simulink model "CameraModel"  (R2024b)
settings: Solver=ode4  StartTime=0.0  StopTime=10.0  FixedStep=0.1  RelTol=1e-3
values from neighbouring files (symbols this model uses):
  cx = W/2    (= 512)    [Camera.m]
  cy = H/2    (= 512)    [Camera.m]
  dt = 0.1    [Camera.m]
  f = W/(2*tan(FOV/2))    [Camera.m]
  H = 1024    [Camera.m]
  I = diag([Ix(5), Iy(5), Iz(5)])    [Camera.m]
  Kd_x = Ix * 2 * zeta * wn    [Camera.m]
  Kd_y = Iy * 2 * zeta * wn    [Camera.m]
  Kd_z = Iz * 2 * zeta * wn    [Camera.m]
  Ki_x = 0.0    (= 0)    [Camera.m]
  Ki_y = 0.0    (= 0)    [Camera.m]
  Ki_z = 0.0    (= 0)    [Camera.m]
  Kp_x = Ix * (wn^2)    [Camera.m]
  Kp_y = Iy * (wn^2)    [Camera.m]
  Kp_z = Iz * (wn^2)    [Camera.m]
  P0 = diag([1e-4, 1e-4, 1e-4, 1e-4, 1e-3, 1e-3, 1e-3])    [Camera.m]
  q_0 = eul2quat([yaw, pitch, roll])    [Camera.m]
  R_c = eul2rotm([yaw, pitch, roll])    [Camera.m]
  sigma = 1    [Camera.m]
  stars = [430.226825035 57.6010327889 -649.101965918 -421.510163393 -579.543487823 -810.977245358 -92.8385341278 591.67322486 632.201742584 -349.161737967 930.305422627 -595.811978564 ... (300 elements, 100x3)]    [Starfield_Test.mat]    (also in generateStars.m = [star_x, star_y, star_z])
  W = 1024    [Camera.m]
  w_0 = [0.01, 0.0, 0.0]'    [Camera.m]
undefined symbols (not defined in the file or in its folder): gray, s_intensity
libraries: slpidlib x3, matrix_library x1, vrlib x1
settings Model: Creator=alejandromunozvazquez  LastModifiedBy=alejandromunozvazquez

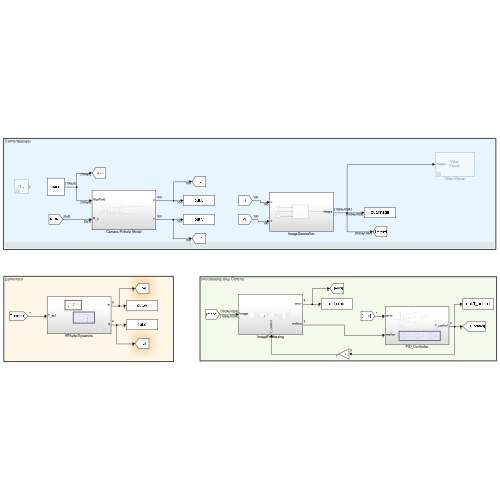
[thumbnail: Simulink's stored preview of the top-level diagram]
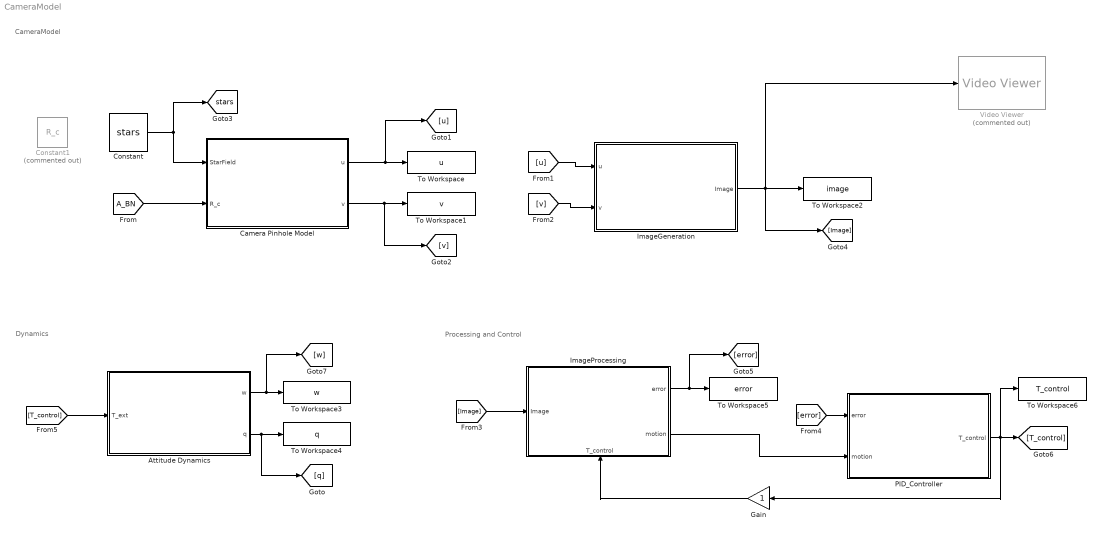
== system CameraModel ==
  note: Processing and Control
  note: Dynamics
  note: CameraModel
  Attitude Dynamics : Subsystem
  Camera Pinhole Model : Subsystem
  Constant : Constant  Value=stars
  Constant1 : Constant  Commented=on  Value=R_c
  Gain : Gain
  ImageGeneration : Subsystem
  ImageProcessing : Subsystem
      settings: PortSchema="{\"entries\":[{\"content\":{\"sides\":[{\"content\":{\"connectorIds\":[\"In1\"]},\"type\":\"ConnectorPlacement.EquallySpacedRectSide\",\"uuid\":\"cefb6310-a581-405a-8101-8623f3d57b98\"},{\"content\":{\"connectorIds\":[\"Out1\",\"Out2\"],\"side\":\"RIGHT\"},\"type\":\"ConnectorPlacement.EquallySpacedRectSide\",\"uuid\":\"16de9d2d-502f-44b2-a135-6b0c6472a31d\"},{\"content\":{\"side\":\"TOP\"},\"type\":\"ConnectorPlacement.EquallySpacedRectSide\",\"uuid\":\"d51e7b6e-a591-4557-adc5-1cc23adf1bf8\"},{\"content\":{\"connectorIds\":[\"In2\"],\"side\":\"BOTTOM\"},\"type\":\"ConnectorPlacement.EquallySpacedRectSide\",\"uuid\":\"ba46090b-2895-4d89-912a-b2ac90d50468\"}]},\"type\":\"ConnectorPlacement.EquallySpacedConnector\",\"uuid\":\"b72943d3-f17b-403e-88fe-0f42ddf20c4f\"}],\"packageUris\":[\"http://schema.mathworks.com/mf0/Connector/R2020b\"],\"version\":\"1.0\"}"
  PID_Controller : Subsystem
  To Workspace : ToWorkspace  VariableName=u  SampleTime=-1
  To Workspace1 : ToWorkspace  VariableName=v  SampleTime=-1
  To Workspace2 : ToWorkspace  VariableName=image  SampleTime=-1
  To Workspace3 : ToWorkspace  VariableName=w  SampleTime=-1
  To Workspace4 : ToWorkspace  VariableName=q  SampleTime=-1
  To Workspace5 : ToWorkspace  VariableName=error  SampleTime=-1
  To Workspace6 : ToWorkspace  VariableName=T_control  SampleTime=-1
  Video Viewer : VideoViewer  Commented=on  colormapValue=gray(256)  FigPos=[336 837 989 604]
  tag scope: stars=global
  wires:
  Attitude Dynamics/1(w) -> [w], To Workspace3/1
  Attitude Dynamics/2(q) -> [q], To Workspace4/1
  Constant/1 -> [stars], Camera Pinhole Model/1(StarField)
  [A_BN] -> Camera Pinhole Model/2(R_c)
  Camera Pinhole Model/1(u) -> [u], To Workspace/1
  Camera Pinhole Model/2(v) -> [v], To Workspace1/1
  [T_control] -> Attitude Dynamics/1(T_ext)
  [u] -> ImageGeneration/1(u)
  [v] -> ImageGeneration/2(v)
  ImageGeneration/1(Image) -> [Image], Video Viewer/1, To Workspace2/1
  [Image] -> ImageProcessing/1(Image)
  ImageProcessing/1(error) -> [error], To Workspace5/1
  [error] -> PID_Controller/1(error)
  PID_Controller/1(T_control) -> Gain/1, [T_control], To Workspace6/1
  ImageProcessing/2(motion) -> PID_Controller/2(motion)
  Gain/1 -> ImageProcessing/2(T_control)

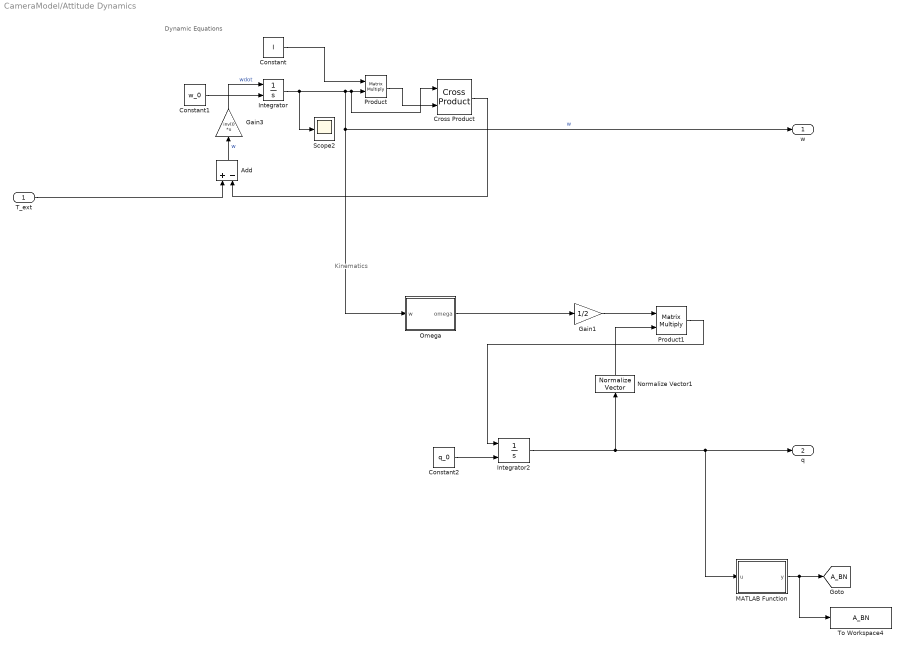
== system CameraModel/Attitude Dynamics ==
  note: Kinematics
  note: Dynamic Equations
  T_ext : Inport
  Add : Sum  Inputs=+-
  Constant : Constant  Value=I
  Constant1 : Constant  Value=w_0
  Constant2 : Constant  Value=q_0
  Cross Product : matrix_library/Cross Product
  Gain1 : Gain  Gain=1/2
  Gain3 : Gain  Gain=inv(I)  Multiplication=Matrix(K*u) (u vector)
  Integrator : Integrator  InitialConditionSource=external
  Integrator2 : Integrator  InitialConditionSource=external
  MATLAB Function : MATLAB Function  TreatAsAtomicUnit=on
  Normalize Vector1 : vrlib/Utilities/Normalize Vector  maxzero=0
  Omega : MATLAB Function  TreatAsAtomicUnit=on
  Product : Product  Multiplication=Matrix(*)
  Product1 : Product  Multiplication=Matrix(*)
  Scope2 : Scope
  To Workspace4 : ToWorkspace  VariableName=A_BN  SampleTime=-1
  w : Outport
  q : Outport  Port=2
  tag scope: A_BN=global
  wires:
  Constant/1 -> Product/1
  Product/1 -> Cross Product/2
  Cross Product/1 -> Add/2
  Integrator/1 -> Scope2/1, Cross Product/1, Product/2, w/1, Omega/1(w)  "w"
  Constant1/1 -> Integrator/2
  T_ext/1 -> Add/1
  Add/1 -> Gain3/1  "w"
  Gain3/1 -> Integrator/1  "wdot"
  Constant2/1 -> Integrator2/2
  Gain1/1 -> Product1/1
  Product1/1 -> Integrator2/1
  Integrator2/1 -> Normalize Vector1/1, MATLAB Function/1(u), q/1
  Normalize Vector1/1 -> Product1/2
  Omega/1(omega) -> Gain1/1
  MATLAB Function/1(y) -> To Workspace4/1, [A_BN]

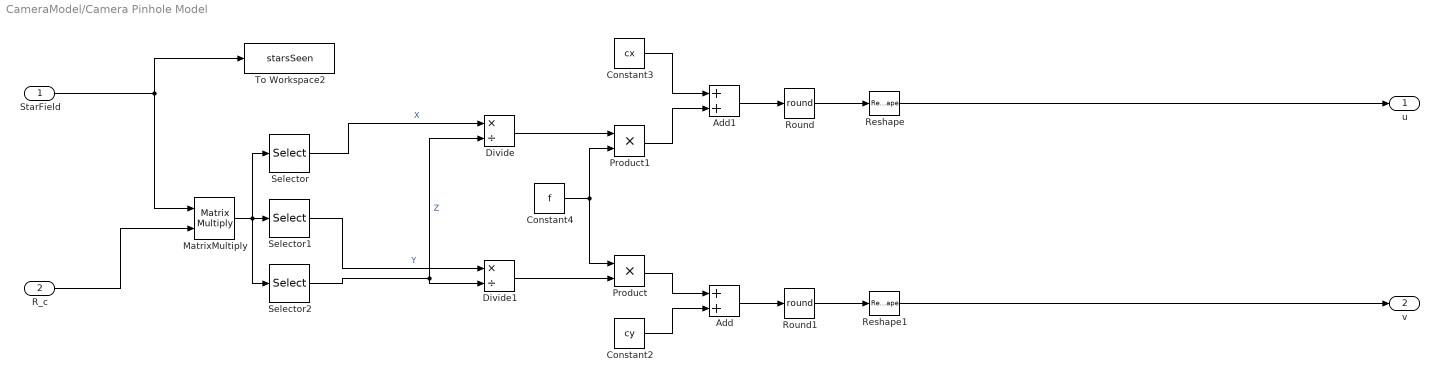
== system CameraModel/Camera Pinhole Model ==
  StarField : Inport
  R_c : Inport  Port=2
  Add : Sum
  Add1 : Sum
  Constant2 : Constant  Value=cy
  Constant3 : Constant  Value=cx
  Constant4 : Constant  Value=f
  Divide : Product  Inputs=*/
  Divide1 : Product  Inputs=*/
  MatrixMultiply : Product  Multiplication=Matrix(*)
  Product : Product
  Product1 : Product
  Reshape : Reshape
  Reshape1 : Reshape
  Round : Rounding  Operator=round
  Round1 : Rounding  Operator=round
  Selector : Selector  NumberOfDimensions=2  InputPortWidth=3  IndexOptions=Select all,Index vector (dialog)  Indices=all,1  OutputSizes=1,1
  Selector1 : Selector  NumberOfDimensions=2  InputPortWidth=3  IndexOptions=Select all,Index vector (dialog)  Indices=all,2  OutputSizes=1,1
  Selector2 : Selector  NumberOfDimensions=2  InputPortWidth=3  IndexOptions=Select all,Index vector (dialog)  Indices=all,3  OutputSizes=1,1
  To Workspace2 : ToWorkspace  VariableName=starsSeen  SampleTime=-1
  u : Outport
  v : Outport  Port=2
  wires:
  Constant2/1 -> Add/2
  R_c/1 -> MatrixMultiply/2
  Round/1 -> Reshape/1
  Divide/1 -> Product1/1
  Product/1 -> Add/1
  Add/1 -> Round1/1
  Selector/1 -> Divide/1  "X"
  Selector1/1 -> Divide1/1  "Y"
  Selector2/1 -> Divide1/2, Divide/2  "Z"
  Add1/1 -> Round/1
  Round1/1 -> Reshape1/1
  MatrixMultiply/1 -> Selector2/1, Selector1/1, Selector/1
  Constant4/1 -> Product/1, Product1/2
  StarField/1 -> MatrixMultiply/1, To Workspace2/1
  Divide1/1 -> Product/2
  Product1/1 -> Add1/2
  Constant3/1 -> Add1/1
  Reshape/1 -> u/1
  Reshape1/1 -> v/1

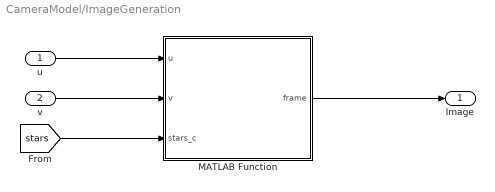
== system CameraModel/ImageGeneration ==
  u : Inport
  v : Inport  Port=2
  MATLAB Function : MATLAB Function  TreatAsAtomicUnit=on
  Image : Outport
  wires:
  u/1 -> MATLAB Function/1(u)
  v/1 -> MATLAB Function/2(v)
  [stars] -> MATLAB Function/3(stars_c)
  MATLAB Function/1(frame) -> Image/1

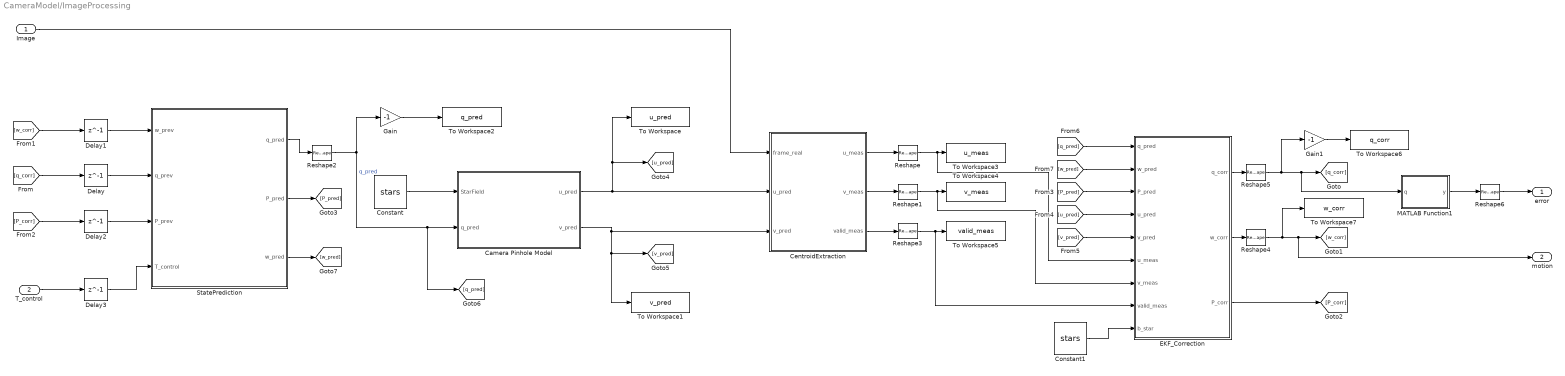
== system CameraModel/ImageProcessing ==
  Image : Inport
  T_control : Inport  Port=2
  Camera Pinhole Model : Subsystem
  CentroidExtraction : MATLAB Function  TreatAsAtomicUnit=on
  Constant : Constant  Value=stars
  Constant1 : Constant  Value=stars
  Delay : Delay  DelayLength=1  InitialCondition=q_0
  Delay1 : Delay  DelayLength=1  InitialCondition=w_0
  Delay2 : Delay  DelayLength=1  InitialCondition=P0
  Delay3 : Delay  DelayLength=1  InitialCondition=[0;0;0]
  EKF_Correction : MATLAB Function  TreatAsAtomicUnit=on
  Gain : Gain  Gain=-1
  Gain1 : Gain  Gain=-1
  MATLAB Function1 : MATLAB Function  TreatAsAtomicUnit=on
  Reshape{,1..6} (7 alike) : Reshape
  StatePrediction : MATLAB Function  TreatAsAtomicUnit=on
  To Workspace : ToWorkspace  VariableName=u_pred  SampleTime=-1
  To Workspace1 : ToWorkspace  VariableName=v_pred  SampleTime=-1
  To Workspace2 : ToWorkspace  VariableName=q_pred  SampleTime=-1
  To Workspace3 : ToWorkspace  VariableName=u_meas  SampleTime=-1
  To Workspace4 : ToWorkspace  VariableName=v_meas  SampleTime=-1
  To Workspace5 : ToWorkspace  VariableName=valid_meas  SampleTime=-1
  To Workspace6 : ToWorkspace  VariableName=q_corr  SampleTime=-1
  To Workspace7 : ToWorkspace  VariableName=w_corr  SampleTime=-1
  error : Outport
  motion : Outport  Port=2
  wires:
  Image/1 -> CentroidExtraction/1(frame_real)
  Delay/1 -> StatePrediction/2(q_prev)
  Delay1/1 -> StatePrediction/1(w_prev)
  StatePrediction/1(q_pred) -> Reshape2/1
  Reshape2/1 -> Gain/1, [q_pred], Camera Pinhole Model/2(q_pred)  "q_pred"
  Constant/1 -> Camera Pinhole Model/1(StarField)
  Camera Pinhole Model/1(u_pred) -> CentroidExtraction/2(u_pred), [u_pred], To Workspace/1
  CentroidExtraction/1(u_meas) -> Reshape/1
  CentroidExtraction/2(v_meas) -> Reshape1/1
  Reshape/1 -> EKF_Correction/6(u_meas), To Workspace3/1
  Reshape1/1 -> EKF_Correction/7(v_meas), To Workspace4/1
  CentroidExtraction/3(valid_meas) -> Reshape3/1
  Reshape3/1 -> EKF_Correction/8(valid_meas), To Workspace5/1
  EKF_Correction/1(q_corr) -> Reshape5/1
  EKF_Correction/3(P_corr) -> [P_corr]
  EKF_Correction/2(w_corr) -> Reshape4/1
  [q_corr] -> Delay/1
  [w_corr] -> Delay1/1
  [P_corr] -> Delay2/1
  Delay2/1 -> StatePrediction/3(P_prev)
  StatePrediction/2(P_pred) -> [P_pred]
  [P_pred] -> EKF_Correction/3(P_pred)
  Constant1/1 -> EKF_Correction/9(b_star)
  Camera Pinhole Model/2(v_pred) -> [v_pred], To Workspace1/1, CentroidExtraction/3(v_pred)
  [v_pred] -> EKF_Correction/5(v_pred)
  [u_pred] -> EKF_Correction/4(u_pred)
  [q_pred] -> EKF_Correction/1(q_pred)
  [w_pred] -> EKF_Correction/2(w_pred)
  StatePrediction/3(w_pred) -> [w_pred]
  Reshape4/1 -> To Workspace7/1, motion/1, [w_corr]
  Reshape5/1 -> Gain1/1, MATLAB Function1/1(q), [q_corr]
  MATLAB Function1/1(y) -> Reshape6/1
  Reshape6/1 -> error/1
  T_control/1 -> Delay3/1
  Delay3/1 -> StatePrediction/4(T_control)
  Gain/1 -> To Workspace2/1
  Gain1/1 -> To Workspace6/1

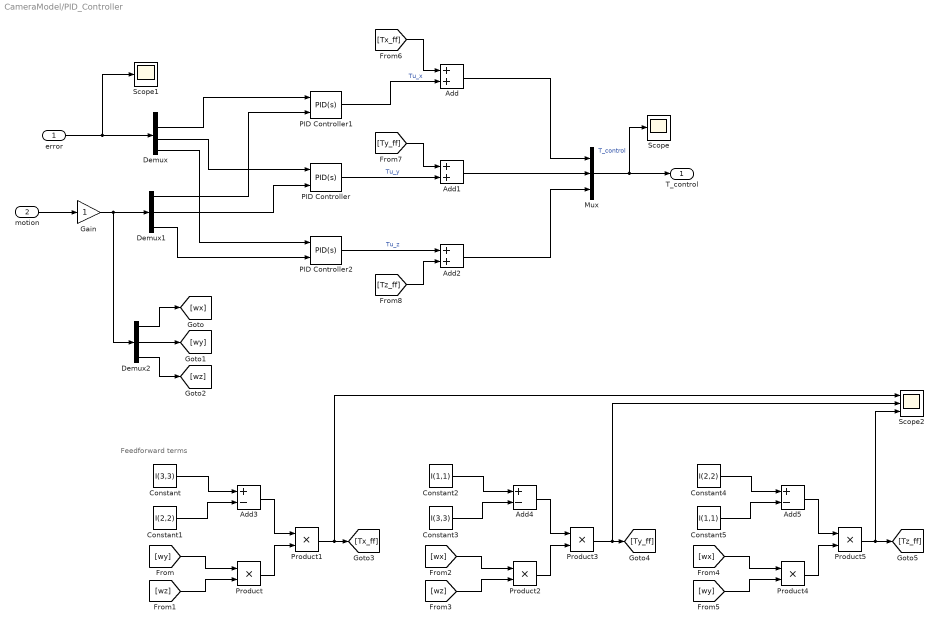
== system CameraModel/PID_Controller ==
  note: Feedforward terms
  error : Inport
  motion : Inport  Port=2
  Add : Sum
  Add1 : Sum
  Add2 : Sum
  Add3 : Sum  Inputs=+-
  Add4 : Sum  Inputs=+-
  Add5 : Sum  Inputs=+-
  Constant : Constant  Value=I(3,3)
  Constant1 : Constant  Value=I(2,2)
  Constant2 : Constant  Value=I(1,1)
  Constant3 : Constant  Value=I(3,3)
  Constant4 : Constant  Value=I(2,2)
  Constant5 : Constant  Value=I(1,1)
  Demux : Demux
  Demux1 : Demux  Outputs=3
  Demux2 : Demux  Outputs=3
  Gain : Gain
  Mux : Mux  Inputs=3
  PID Controller : slpidlib/PID Controller  Controller=PID  Form=Parallel  TimeDomain=Continuous-time  UseExternalTs=off  SampleTime=-1  IntegratorMethod=Forward Euler  FilterMethod=Forward Euler  ControllerParametersSource=internal  P=Kp_y  I=Ki_y  UseKiTs=off  D=Kd_y  UseExternalDerivativeSource=on  N=10  UseFilter=on  TunerSelectOption=Transfer Function Based (PID Tuner App)  InitialConditionSource=internal  InitialConditionForIntegrator=0  InitialConditionForFilter=0  DifferentiatorICPrevScaledInput=0  ExternalReset=none  TrackingMode=off  Kt=1  LimitOutput=off  SatLimitsSource=internal  UpperSaturationLimit=inf  LowerSaturationLimit=-inf  LinearizeAsGain=on  AntiWindupMode=none  Kb=1  LimitIntegrator=off  UpperIntegratorSaturationLimit=inf  LowerIntegratorSaturationLimit=-inf  POutMin=[]  POutMax=[]  IOutMin=[]  IOutMax=[]  DOutMin=[]  DOutMax=[]  NOutMin=[]  NOutMax=[]  SumOutMin=[]  SumOutMax=[]  SaturationOutMin=[]  SaturationOutMax=[]  PParamMin=[]  PParamMax=[]  IParamMin=[]  IParamMax=[]  DParamMin=[]  DParamMax=[]  NParamMin=[]  NParamMax=[]  KbParamMin=[]  KbParamMax=[]  KtParamMin=[]  KtParamMax=[]  KbOutMin=[]  KbOutMax=[]  KtOutMin=[]  KtOutMax=[]  IntegratorOutMin=[]  IntegratorOutMax=[]  FilterOutMin=[]  FilterOutMax=[]  SumI1OutMin=[]  SumI1OutMax=[]  SumI2OutMin=[]  SumI2OutMax=[]  SumI3OutMin=[]  SumI3OutMax=[]  SumI4OutMin=[]  SumI4OutMax=[]  SumDOutMin=[]  SumDOutMax=[]  DifferentiatorOutMin=[]  DifferentiatorOutMax=[]  FilterDiffOutCoefMin=[]  FilterDiffOutCoefMax=[]  ReciprocalOutMin=[]  ReciprocalOutMax=[]  SumDenOutMin=[]  SumDenOutMax=[]  SumNumOutMin=[]  SumNumOutMax=[]  DivideOutMin=[]  DivideOutMax=[]  UdiffTsProdOutMin=[]  UdiffTsProdOutMax=[]  NTsProdOutMin=[]  NTsProdOutMax=[]  UintegralTsProdOutMin=[]  UintegralTsProdOutMax=[]  UngainTsProdOutMin=[]  UngainTsProdOutMax=[]  ClampingZeroOutDataTypeStr=Inherit: Inherit via back propagation  ClampingZeroOutMin=[]  ClampingZeroOutMax=[]  FilterDenConstantOutDataTypeStr=Inherit: Inherit via back propagation  FilterDenConstantOutMin=[]  FilterDenConstantOutMax=[]  PCopyOutDataTypeStr=Inherit: Inherit via back propagation  PCopyOutMin=[]  PCopyOutMax=[]  NCopyOutDataTypeStr=Inherit: Inherit via back propagation  NCopyOutMin=[]  NCopyOutMax=[]  IntegratorContinuousStateAttributes=''  IntegratorStateMustResolveToSignalObject=off  IntegratorRTWStateStorageClass=Auto  FilterContinuousStateAttributes=''  FilterStateMustResolveToSignalObject=off  FilterRTWStateStorageClass=Auto  ParallelPVariant=InternalParameters  IdealPVariant=Disabled  IVariant=InternalParameters  DVariant=InternalParameters  IntegratorVariant=Continuous  SatVariant=Disabled  AWVariant=Passthrough  PCopyVariant=Disabled  TRVariant=Disabled  FdbkBlocksVariant=Forward  IdealPFdbkVariant=Disabled  SatFdbkVariant=Disabled  DerivativeFilterVariant=ContFilterOnly  NVariant=InternalParameters  NCopyVariant=Disabled  FilterICVariant=InternalICsFilter  IntegratorICVariant=InternalICs  ExternalResetVariant=Disabled  TRSumVariant=Passthrough  SumFdbkVariant=Disabled  SumVariant=Sum_PID  TsampFilterVariant=InternalTs  TsampNgainVariant=Passthrough  TsampIntegralVariant=Disabled_SignalSpec  ExternalSaturationOutDataTypeStr=Inherit: Same as second input  DerivativeSourceVariant=ExternalYdot  PreIntVariant=InternalPreInt
  PID Controller1 : slpidlib/PID Controller  Controller=PID  Form=Parallel  TimeDomain=Continuous-time  UseExternalTs=off  SampleTime=-1  IntegratorMethod=Forward Euler  FilterMethod=Forward Euler  ControllerParametersSource=internal  P=Kp_x  I=Ki_x  UseKiTs=off  D=Kd_x  UseExternalDerivativeSource=on  N=10  UseFilter=on  TunerSelectOption=Transfer Function Based (PID Tuner App)  InitialConditionSource=internal  InitialConditionForIntegrator=0  InitialConditionForFilter=0  DifferentiatorICPrevScaledInput=0  ExternalReset=none  TrackingMode=off  Kt=1  LimitOutput=off  SatLimitsSource=internal  UpperSaturationLimit=inf  LowerSaturationLimit=-inf  LinearizeAsGain=on  AntiWindupMode=none  Kb=1  LimitIntegrator=off  UpperIntegratorSaturationLimit=inf  LowerIntegratorSaturationLimit=-inf  POutMin=[]  POutMax=[]  IOutMin=[]  IOutMax=[]  DOutMin=[]  DOutMax=[]  NOutMin=[]  NOutMax=[]  SumOutMin=[]  SumOutMax=[]  SaturationOutMin=[]  SaturationOutMax=[]  PParamMin=[]  PParamMax=[]  IParamMin=[]  IParamMax=[]  DParamMin=[]  DParamMax=[]  NParamMin=[]  NParamMax=[]  KbParamMin=[]  KbParamMax=[]  KtParamMin=[]  KtParamMax=[]  KbOutMin=[]  KbOutMax=[]  KtOutMin=[]  KtOutMax=[]  IntegratorOutMin=[]  IntegratorOutMax=[]  FilterOutMin=[]  FilterOutMax=[]  SumI1OutMin=[]  SumI1OutMax=[]  SumI2OutMin=[]  SumI2OutMax=[]  SumI3OutMin=[]  SumI3OutMax=[]  SumI4OutMin=[]  SumI4OutMax=[]  SumDOutMin=[]  SumDOutMax=[]  DifferentiatorOutMin=[]  DifferentiatorOutMax=[]  FilterDiffOutCoefMin=[]  FilterDiffOutCoefMax=[]  ReciprocalOutMin=[]  ReciprocalOutMax=[]  SumDenOutMin=[]  SumDenOutMax=[]  SumNumOutMin=[]  SumNumOutMax=[]  DivideOutMin=[]  DivideOutMax=[]  UdiffTsProdOutMin=[]  UdiffTsProdOutMax=[]  NTsProdOutMin=[]  NTsProdOutMax=[]  UintegralTsProdOutMin=[]  UintegralTsProdOutMax=[]  UngainTsProdOutMin=[]  UngainTsProdOutMax=[]  ClampingZeroOutDataTypeStr=Inherit: Inherit via back propagation  ClampingZeroOutMin=[]  ClampingZeroOutMax=[]  FilterDenConstantOutDataTypeStr=Inherit: Inherit via back propagation  FilterDenConstantOutMin=[]  FilterDenConstantOutMax=[]  PCopyOutDataTypeStr=Inherit: Inherit via back propagation  PCopyOutMin=[]  PCopyOutMax=[]  NCopyOutDataTypeStr=Inherit: Inherit via back propagation  NCopyOutMin=[]  NCopyOutMax=[]  IntegratorContinuousStateAttributes=''  IntegratorStateMustResolveToSignalObject=off  IntegratorRTWStateStorageClass=Auto  FilterContinuousStateAttributes=''  FilterStateMustResolveToSignalObject=off  FilterRTWStateStorageClass=Auto  ParallelPVariant=InternalParameters  IdealPVariant=Disabled  IVariant=InternalParameters  DVariant=InternalParameters  IntegratorVariant=Continuous  SatVariant=Disabled  AWVariant=Passthrough  PCopyVariant=Disabled  TRVariant=Disabled  FdbkBlocksVariant=Forward  IdealPFdbkVariant=Disabled  SatFdbkVariant=Disabled  DerivativeFilterVariant=ContFilterOnly  NVariant=InternalParameters  NCopyVariant=Disabled  FilterICVariant=InternalICsFilter  IntegratorICVariant=InternalICs  ExternalResetVariant=Disabled  TRSumVariant=Passthrough  SumFdbkVariant=Disabled  SumVariant=Sum_PID  TsampFilterVariant=InternalTs  TsampNgainVariant=Passthrough  TsampIntegralVariant=Disabled_SignalSpec  ExternalSaturationOutDataTypeStr=Inherit: Same as second input  DerivativeSourceVariant=ExternalYdot  PreIntVariant=InternalPreInt
  PID Controller2 : slpidlib/PID Controller  Controller=PID  Form=Parallel  TimeDomain=Continuous-time  UseExternalTs=off  SampleTime=-1  IntegratorMethod=Forward Euler  FilterMethod=Forward Euler  ControllerParametersSource=internal  P=Kp_z  I=Ki_z  UseKiTs=off  D=Kd_z  UseExternalDerivativeSource=on  N=10  UseFilter=on  TunerSelectOption=Transfer Function Based (PID Tuner App)  InitialConditionSource=internal  InitialConditionForIntegrator=0  InitialConditionForFilter=0  DifferentiatorICPrevScaledInput=0  ExternalReset=none  TrackingMode=off  Kt=1  LimitOutput=off  SatLimitsSource=internal  UpperSaturationLimit=inf  LowerSaturationLimit=-inf  LinearizeAsGain=on  AntiWindupMode=none  Kb=1  LimitIntegrator=off  UpperIntegratorSaturationLimit=inf  LowerIntegratorSaturationLimit=-inf  POutMin=[]  POutMax=[]  IOutMin=[]  IOutMax=[]  DOutMin=[]  DOutMax=[]  NOutMin=[]  NOutMax=[]  SumOutMin=[]  SumOutMax=[]  SaturationOutMin=[]  SaturationOutMax=[]  PParamMin=[]  PParamMax=[]  IParamMin=[]  IParamMax=[]  DParamMin=[]  DParamMax=[]  NParamMin=[]  NParamMax=[]  KbParamMin=[]  KbParamMax=[]  KtParamMin=[]  KtParamMax=[]  KbOutMin=[]  KbOutMax=[]  KtOutMin=[]  KtOutMax=[]  IntegratorOutMin=[]  IntegratorOutMax=[]  FilterOutMin=[]  FilterOutMax=[]  SumI1OutMin=[]  SumI1OutMax=[]  SumI2OutMin=[]  SumI2OutMax=[]  SumI3OutMin=[]  SumI3OutMax=[]  SumI4OutMin=[]  SumI4OutMax=[]  SumDOutMin=[]  SumDOutMax=[]  DifferentiatorOutMin=[]  DifferentiatorOutMax=[]  FilterDiffOutCoefMin=[]  FilterDiffOutCoefMax=[]  ReciprocalOutMin=[]  ReciprocalOutMax=[]  SumDenOutMin=[]  SumDenOutMax=[]  SumNumOutMin=[]  SumNumOutMax=[]  DivideOutMin=[]  DivideOutMax=[]  UdiffTsProdOutMin=[]  UdiffTsProdOutMax=[]  NTsProdOutMin=[]  NTsProdOutMax=[]  UintegralTsProdOutMin=[]  UintegralTsProdOutMax=[]  UngainTsProdOutMin=[]  UngainTsProdOutMax=[]  ClampingZeroOutDataTypeStr=Inherit: Inherit via back propagation  ClampingZeroOutMin=[]  ClampingZeroOutMax=[]  FilterDenConstantOutDataTypeStr=Inherit: Inherit via back propagation  FilterDenConstantOutMin=[]  FilterDenConstantOutMax=[]  PCopyOutDataTypeStr=Inherit: Inherit via back propagation  PCopyOutMin=[]  PCopyOutMax=[]  NCopyOutDataTypeStr=Inherit: Inherit via back propagation  NCopyOutMin=[]  NCopyOutMax=[]  IntegratorContinuousStateAttributes=''  IntegratorStateMustResolveToSignalObject=off  IntegratorRTWStateStorageClass=Auto  FilterContinuousStateAttributes=''  FilterStateMustResolveToSignalObject=off  FilterRTWStateStorageClass=Auto  ParallelPVariant=InternalParameters  IdealPVariant=Disabled  IVariant=InternalParameters  DVariant=InternalParameters  IntegratorVariant=Continuous  SatVariant=Disabled  AWVariant=Passthrough  PCopyVariant=Disabled  TRVariant=Disabled  FdbkBlocksVariant=Forward  IdealPFdbkVariant=Disabled  SatFdbkVariant=Disabled  DerivativeFilterVariant=ContFilterOnly  NVariant=InternalParameters  NCopyVariant=Disabled  FilterICVariant=InternalICsFilter  IntegratorICVariant=InternalICs  ExternalResetVariant=Disabled  TRSumVariant=Passthrough  SumFdbkVariant=Disabled  SumVariant=Sum_PID  TsampFilterVariant=InternalTs  TsampNgainVariant=Passthrough  TsampIntegralVariant=Disabled_SignalSpec  ExternalSaturationOutDataTypeStr=Inherit: Same as second input  DerivativeSourceVariant=ExternalYdot  PreIntVariant=InternalPreInt
  Product{,1..5} (6 alike) : Product
  Scope : Scope
  Scope1 : Scope
  Scope2 : Scope  NumInputPorts=3
  T_control : Outport
  wires:
  error/1 -> Scope1/1, Demux/1
  Demux/3 -> PID Controller/1
  Demux/2 -> PID Controller1/1
  PID Controller/1 -> Add1/2  "Tu_y"
  PID Controller1/1 -> Add/2  "Tu_x"
  Demux/4 -> PID Controller2/1
  PID Controller2/1 -> Add2/1  "Tu_z"
  Mux/1 -> T_control/1, Scope/1  "T_control"
  motion/1 -> Gain/1
  Demux1/1 -> PID Controller1/2
  Gain/1 -> Demux2/1, Demux1/1
  Demux1/3 -> PID Controller2/2
  Demux1/2 -> PID Controller/2
  Demux2/1 -> [wx]
  Demux2/2 -> [wy]
  Demux2/3 -> [wz]
  Constant1/1 -> Add3/2
  Constant/1 -> Add3/1
  [wy] -> Product/1
  [wz] -> Product/2
  Add3/1 -> Product1/1
  Product/1 -> Product1/2
  Product1/1 -> Scope2/1, [Tx_ff]
  Product3/1 -> Scope2/2, [Ty_ff]
  Product2/1 -> Product3/2
  Add4/1 -> Product3/1
  [wz] -> Product2/2
  [wx] -> Product2/1
  Constant2/1 -> Add4/1
  Constant3/1 -> Add4/2
  Constant5/1 -> Add5/2
  Constant4/1 -> Add5/1
  [wx] -> Product4/1
  [wy] -> Product4/2
  Add5/1 -> Product5/1
  Product4/1 -> Product5/2
  Product5/1 -> Scope2/3, [Tz_ff]
  [Tx_ff] -> Add/1
  [Ty_ff] -> Add1/1
  [Tz_ff] -> Add2/2
  Add/1 -> Mux/1
  Add1/1 -> Mux/2
  Add2/1 -> Mux/3

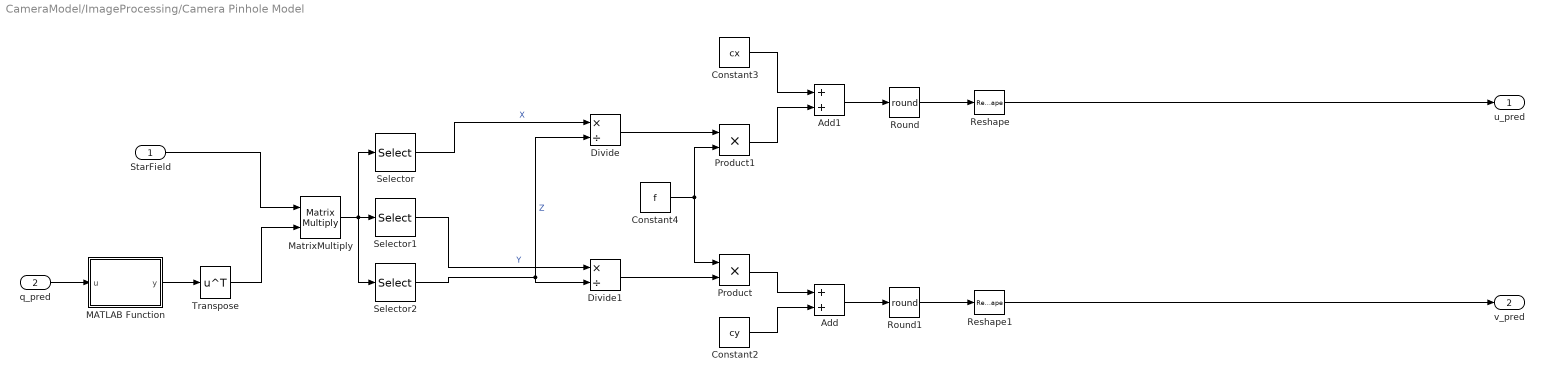
== system CameraModel/ImageProcessing/Camera Pinhole Model ==
  StarField : Inport
  q_pred : Inport  Port=2
  Add : Sum
  Add1 : Sum
  Constant2 : Constant  Value=cy
  Constant3 : Constant  Value=cx
  Constant4 : Constant  Value=f
  Divide : Product  Inputs=*/
  Divide1 : Product  Inputs=*/
  MATLAB Function : MATLAB Function  TreatAsAtomicUnit=on
  MatrixMultiply : Product  Multiplication=Matrix(*)
  Product : Product
  Product1 : Product
  Reshape : Reshape
  Reshape1 : Reshape
  Round : Rounding  Operator=round
  Round1 : Rounding  Operator=round
  Selector : Selector  NumberOfDimensions=2  InputPortWidth=3  IndexOptions=Select all,Index vector (dialog)  Indices=all,1  OutputSizes=1,1
  Selector1 : Selector  NumberOfDimensions=2  InputPortWidth=3  IndexOptions=Select all,Index vector (dialog)  Indices=all,2  OutputSizes=1,1
  Selector2 : Selector  NumberOfDimensions=2  InputPortWidth=3  IndexOptions=Select all,Index vector (dialog)  Indices=all,3  OutputSizes=1,1
  Transpose : Math  Operator=transpose
  u_pred : Outport
  v_pred : Outport  Port=2
  wires:
  Constant2/1 -> Add/2
  q_pred/1 -> MATLAB Function/1(u)
  Round/1 -> Reshape/1
  Divide/1 -> Product1/1
  Product/1 -> Add/1
  Add/1 -> Round1/1
  Selector/1 -> Divide/1  "X"
  Selector1/1 -> Divide1/1  "Y"
  Selector2/1 -> Divide1/2, Divide/2  "Z"
  Add1/1 -> Round/1
  Round1/1 -> Reshape1/1
  MatrixMultiply/1 -> Selector2/1, Selector1/1, Selector/1
  Constant4/1 -> Product/1, Product1/2
  StarField/1 -> MatrixMultiply/1
  Divide1/1 -> Product/2
  Product1/1 -> Add1/2
  Constant3/1 -> Add1/1
  Reshape/1 -> u_pred/1
  Reshape1/1 -> v_pred/1
  MATLAB Function/1(y) -> Transpose/1
  Transpose/1 -> MatrixMultiply/2

== matlab function CameraModel/ImageProcessing/MATLAB Function1 ==
  data: q input; y output; q_0 parameter
function y = fcn(q, q_0)

    q_0 = q_0(:) / norm(q_0);
    q   = q(:)   / norm(q);

    % Inverso = conjugado para cuaterniones unitarios
    q_inv = [q_0(1); -q_0(2); -q_0(3); -q_0(4)];

    % Producto cuaterniónico manual: q_err = q_inv ⊗ q
    % Convenio [w, x, y, z]
    w1=q_inv(1); x1=q_inv(2); y1=q_inv(3); z1=q_inv(4);
    w2=q(1);     x2=q(2);     y2=q(3);     z2=q(4);

    q_err = [ w1*w2 - x1*x2 - y1*y2 - z1*z2;
              w1*x2 + x1*w2 + y1*z2 - z1*y2;
              w1*y2 - x1*z2 + y1*w2 + z1*x2;
              w1*z2 + x1*y2 - y1*x2 + z1*w2 ];

    % Ángulos de Euler del error
    %y = quat2eul(q_err');
    y = [q_err(1); q_err(2); q_err(3); q_err(4)];
end

== matlab function CameraModel/Attitude Dynamics/Omega ==
  data: w input; omega output size=[4,4]
function omega = fcn(w)

omega = zeros(4,4);
wx = w(1);
wy = w(2);
wz = w(3);



omega = [0  -wx -wy -wz;
     wx  0   wz -wy;
     wy -wz  0   wx;
     wz  wy -wx  0];

end

== matlab function CameraModel/ImageGeneration/MATLAB Function ==
  data: u input; frame output; v input; stars_c input; W parameter; H parameter; sigma parameter; s_intensity parameter
function frame = fcn(u, v, stars_c, W, H, sigma, s_intensity)
    
    frame = zeros(H, W, 'uint8');

    N = length(u);
    % I_0 = zeros(length(s_intensity),1);
    % n = 5;

    for i = 1:N
        if stars_c(i,3) > 0
            if (u(i)>0 && u(i)<=W) && (v(i)>0 && v(i)<=H)
                
                frame(v(i),u(i)) = 255;
                
                % Para posteriormente dar realismo a la imagen
                % [X, Y] = meshgrid(u(i)-n : u(i)+n, v(i)-n : v(i)+n);
                % I_0(i) = s_intensity(i)*1000;
                % 
                % % Aplicar la función Gaussiana bidimensional
                % if (u(i)>n && u(i)<W-n) && (v(i)>n && v(i)<H-n)
                %     frame(v(i)-n:v(i)+n,u(i)-n:u(i)+n) = I_0(i) * exp(-((X - u(i)).^2 + (Y - v(i)).^2) / (2 * sigma^2));
                % end

            end
        end
    end
end

== matlab function CameraModel/Attitude Dynamics/MATLAB Function ==
  data: u input; y output
function y = fcn(u)

y = quat2rotm([u(1) u(2) u(3) u(4)]);

== matlab function CameraModel/ImageProcessing/StatePrediction ==
  settings: updateMethod=DISCRETE  sampleTime=0.1
  data: w_prev input; q_prev input; P_prev input; dt parameter; q_pred output size=[4, 1]; P_pred output; w_pred output; T_control input; I parameter
function [q_pred, P_pred, w_pred] = fcn(w_prev, q_prev, P_prev, dt, T_control, I)
    %Variables
    q_prev = q_prev(:);
    T_control = T_control(:);
    w_pred = zeros(3,1);
    
    % Auxiliary variables
    wx = w_prev(1); wy = w_prev(2); wz = w_prev(3);
    W_prev = [0 -wx -wy -wz; wx 0 wz -wy; wy -wz 0 wx; wz wy -wx 0]; %Convenio estandar
    

    sigma_q = 1e-6;  % Ruido en cuaternión (ajustar según giróscopo)
    sigma_w = 1e-3;  % Ruido en bias (random walk)
    Q_noise = diag([sigma_q*ones(1,4), sigma_w*ones(1,3)]);

    % Transition matrix
    w_n = norm(w_prev);

    if w_n < 1e-5
        Q_tran = eye(4) + (dt/2)*W_prev;
    else
        Q_tran = cos(w_n*dt/2)*eye(4) + (1/w_n)*sin(w_n*dt/2)*W_prev;
    end
    % Jacobian state transition matrix
    q0 = q_prev(1); q1 = q_prev(2); q2 = q_prev(3); q3 = q_prev(4);
    E_prev = (dt/2)*[-q1 -q2 -q3; q0 -q3 q2; q3 q0 -q1; -q2 q1 q0]; %Convenio estandar

    
    phi_prev = [Q_tran E_prev; zeros(3,4) eye(3)];         

    % Kalman Filter
    q_pred = Q_tran*q_prev; 
    q_pred = q_pred * (1/norm(q_pred));
    P_pred = phi_prev*P_prev*phi_prev' + Q_noise;  

    Ix = I(1,1);
    Iy = I(2,2);
    Iz = I(3,3);

    % Ecuaciones de Euler con torque de control
    dwx = (T_control(1) - (Iz - Iy)*wy*wz) / Ix;
    dwy = (T_control(2) - (Ix - Iz)*wx*wz) / Iy;
    dwz = (T_control(3) - (Iy - Ix)*wx*wy) / Iz;
    
    w_pred(1) = w_prev(1) + dwx * dt;
    w_pred(2) = w_prev(2) + dwy * dt;
    w_pred(3) = w_prev(3) + dwz * dt;


end

== matlab function CameraModel/ImageProcessing/Camera Pinhole Model/MATLAB Function ==
  data: u input; y output
function y = fcn(u)

y = quat2rotm([u(1) u(2) u(3) u(4)]);

== matlab function CameraModel/ImageProcessing/CentroidExtraction ==
  data: frame_real input; u_meas output; u_pred input; v_pred input; v_meas output; valid_meas output; W parameter; H parameter
function [u_meas, v_meas, valid_meas] = fcn(frame_real, u_pred, v_pred, W, H)

    % Parameters
    W_win = 10;
    N = length(u_pred);

    %Initialization
    u_meas = zeros(N,1);
    v_meas = zeros(N,1);
    valid_meas = false(N,1);

    frame_d = double(frame_real);

    for i=1:N
        
        uc = round(u_pred(i));
        vc = round(v_pred(i));

        if uc<1 || uc>W || vc<1 || vc>H
            continue;
        end

        u_min = max(1, uc-W_win);
        u_max = min(W, uc+W_win);
        v_min = max(1, vc-W_win);
        v_max = min(H, vc+W_win);

        win = frame_d(v_min:v_max, u_min:u_max);

        S = sum(win(:));

        if S>0
            u_coords = u_min:u_max;
            v_coords = (v_min:v_max)';

            u_meas(i) = (v_coords*0+1)'*(win*u_coords') / S;
            v_meas(i) = (v_coords'*win*ones(size(win,2),1)) / S;

            valid_meas(i) = true;
        end
    end
end

== matlab function CameraModel/ImageProcessing/EKF_Correction ==
  data: q_pred input; w_pred input; P_pred input; q_corr output; u_pred input; v_pred input; u_meas input; v_meas input; valid_meas input; b_star input; w_corr output; P_corr output; W parameter; H parameter; f parameter
function [q_corr, w_corr, P_corr] = fcn(q_pred, w_pred, P_pred, u_pred, v_pred, u_meas, v_meas, valid_meas, b_star, W, H, f)

    % --- Forzar dimensiones ---
    q_pred     = q_pred(:);
    w_pred     = w_pred(:);
    u_pred     = u_pred(:);
    v_pred     = v_pred(:);
    u_meas     = u_meas(:);
    v_meas     = v_meas(:);
    valid_meas = logical(valid_meas(:));

    % --- Pre-declarar salidas ---
    q_corr = zeros(4,1);
    w_corr = zeros(3,1);
    P_corr = zeros(7,7);

    % --- Constantes ---
    persistent R_noise
    if isempty(R_noise), R_noise = 10.0; end

    N      = length(u_pred);
    X_base = [q_pred; w_pred];

    % ----------------------------------------------------------------
    % 1. Innovación dz y R_mat
    % ----------------------------------------------------------------
    dz    = zeros(2*N, 1);
    R_vec = ones(2*N, 1) * R_noise;

    for k = 1:N
        if valid_meas(k)
            dz(2*k-1) = u_meas(k) - u_pred(k);
            dz(2*k)   = v_meas(k) - v_pred(k);
        else
            R_vec(2*k-1) = 1e9;
            R_vec(2*k)   = 1e9;
        end
    end
    R_mat = diag(R_vec);

    % ----------------------------------------------------------------
    % 2. Jacobiano analítico
    % ----------------------------------------------------------------
    H_mat  = zeros(2*N, 7);
    A_base = quat2rotm(q_pred');
    pos    = (A_base * b_star')';
    q0 = q_pred(1); q1 = q_pred(2); q2 = q_pred(3); q3 = q_pred(4);

    for k = 1:N
        if valid_meas(k) && abs(pos(k,3)) > 1e-6
            bx = b_star(k,1); by = b_star(k,2); bz = b_star(k,3);
            xk = pos(k,1);    yk = pos(k,2);    zk = pos(k,3);

            dxdq = 2*[q0*bx - q3*by + q2*bz,  q1*bx + q2*by + q3*bz, ...
                      q2*bx - q1*by + q0*bz,  q3*bx - q0*by - q1*bz];
            dydq = 2*[q0*by + q3*bx - q1*bz,  q1*by - q2*bx - q0*bz, ...
                      q2*by + q1*bx + q3*bz,  q3*by + q0*bx - q2*bz];
            dzdq = 2*[q0*bz - q2*bx + q1*by,  q1*bz + q3*bx + q0*by, ...
                      q2*bz + q3*by - q0*bx,  q3*bz - q1*bx - q2*by];

            H_mat(2*k-1, 1:4) = f/zk * dxdq - (f*xk/zk^2) * dzdq;
            H_mat(2*k,   1:4) = f/zk * dydq - (f*yk/zk^2) * dzdq;
        end
    end

    % ----------------------------------------------------------------
    % 3. Ecuaciones del EKF
    % ----------------------------------------------------------------
    S      = H_mat * P_pred * H_mat' + R_mat;
    S = S + 1e-8 * eye(size(S,1));
    K      = (P_pred * H_mat') / S;

    X_corr = X_base + K * dz;
    q_corr = X_corr(1:4);
    q_corr = q_corr * (1/norm(q_corr));
    w_corr = X_corr(5:7);

    IKH    = eye(7) - K * H_mat;
    P_corr = IKH * P_pred * IKH' + K * R_mat * K';
    P_corr = (P_corr + P_corr') * 0.5;

    % Después del Jacobiano
    if any(isnan(H_mat(:))), disp('NaN en H_mat'); end
    
    % Después de S
    if any(isnan(S(:))), disp('NaN en S'); end
    if rcond(S) < 1e-15,  disp('S singular, rcond='), disp(rcond(S)); end
    
    % Después de K
    if any(isnan(K(:))), disp('NaN en K'); end
end
